simulink library "ammclib_bam_s32k11x"  (Simulink 9.0)
settings: Solver=ode45  StartTime=0.0  StopTime=10.0  RelTol=1e-3
undefined symbols (not defined in the file): f16A1, f16A2, f16B0, f16B1, f16B2, f16C1, f16CC1, f16CC1sc, f16CC1sc_D, f16CC1sc_Q, f16CC1scD, f16CC1scQ, f16CC2, f16CC2sc, f16CC2sc_D, f16CC2sc_Q, f16CC2scD, f16CC2scQ, f16DerivGain, f16EGain, f16FiltCoef, f16HystOff, f16HystOn, f16IGain, f16IntegGain, f16IntegGainFW, f16IntegGainQ, f16Kd, f16Kq, f16Limit, f16LowerLim, f16LowerLimit_D, f16LowerLimit_Q, f16ModIndex, f16OutValOff, f16OutValOn, f16PropGain, f16PropGainFW, f16PropGainQ, f16RampDown, f16RampUp, f16UGain, f16UpperLim, f16UpperLimit, f16UpperLimit_D, f16UpperLimit_Q, f16WIGain, f32A1, f32A2, f32B0, f32B1, f32B2, f32C1, f32CC1, f32CC1sc, f32CC1sc_D, f32CC1sc_Q, f32CC1scD, f32CC1scQ, f32CC2 ... (+71)
(part 1 of 7)
settings Model: Creator=STSP001  LastModifiedBy=nxf35375

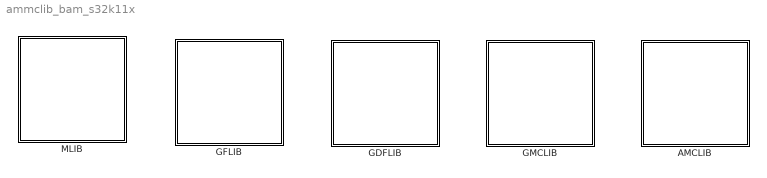
== system ammclib_bam_s32k11x ==
  AMCLIB : Subsystem
  GDFLIB : Subsystem
  GFLIB : Subsystem
  GMCLIB : Subsystem
  MLIB : Subsystem

== system ammclib_bam_s32k11x/AMCLIB ==
  bam_f16 : Subsystem
  bam_f32 : Subsystem

== system ammclib_bam_s32k11x/GDFLIB ==
  bam_f16 : Subsystem
  bam_f32 : Subsystem

== system ammclib_bam_s32k11x/GFLIB ==
  bam_f16 : Subsystem
  bam_f32 : Subsystem

== system ammclib_bam_s32k11x/GMCLIB ==
  bam_f16 : Subsystem
  bam_f32 : Subsystem

== system ammclib_bam_s32k11x/MLIB ==
  bam_f16 : Subsystem
  bam_f32 : Subsystem
  bam_f32f16f16 : Subsystem

== system ammclib_bam_s32k11x/AMCLIB/bam_f16 ==
  AMCLIB_BemfObsrvDQ_F16 : Subsystem  mask(AMCLIB_BemfObsrvDQ_F16){f16IGain=f16IGain, f16UGain=f16UGain, f16WIGain=f16WIGain, f16EGain=f16EGain, s16Shift=s16Shift, f16CC1sc_D=f16CC1sc_D, f16CC1sc_Q=f16CC1sc_Q, f16CC2sc_D=f16CC2sc_D, f16CC2sc_Q=f16CC2sc_Q, f16UpperLimit_D=f16UpperLimit_D, f16UpperLimit_Q=f16UpperLimit_Q, f16LowerLimit_D=f16LowerLimit_D, f16LowerLimit_Q=f16LowerLimit_Q, u16NShift=u16NShift}
      mask help: Bit accurate model of back-EMF observer DQ in 16-bit fixed-point implementation.
      mask init:
      | pos = get_param(gcb, 'Position');width = pos(3) - pos(1); height = pos(4) - pos(2);tX=width/2;tY=height*0.9;
      mask Display: color('black');port_label('input',1,'f16IAB_A');port_label('input',2,'f16IAB_B');port_label('input',3,'f16UAB_A');port_label('input',4,'f16UAB_B');port_label('input',5,'f16Velocity');port_label('input',6,'f16Phase');port_label('output',1,'f16pOutPhaseErr');port_label('output',2,'f16pOutEObsrv_D');port_label('output',3,'f16pOutEObsrv_Q');color('black');disp('AMCLIB_BemfObsrvDQ_F16');color('blue');text(tX,tY, 'BAM', 'horizontalAlignment', 'center');
  AMCLIB_CurrentLoop_F16 : Subsystem  mask(AMCLIB_CurrentLoop_F16){f16CC1scD=f16CC1scD, f16CC2scD=f16CC2scD, u16NShiftD=u16NShiftD, f16CC1scQ=f16CC1scQ, f16CC2scQ=f16CC2scQ, u16NShiftQ=u16NShiftQ}
      mask help: Bit accurate model of the current loop algorithm for a PMSM in 16-bit fixed-point implementation.
      mask init:
      | pos = get_param(gcb, 'Position');width = pos(3) - pos(1); height = pos(4) - pos(2);tX=width/2;tY=height*0.9;
      mask Display: color('black');port_label('input',1,'f16UDcBus');port_label('input',2,'f16IDReq');port_label('input',3,'f16IQReq');port_label('input',4,'f16IDFbck');port_label('input',5,'f16IQFbck');port_label('output',1,'pOutUDReq');port_label('output',2,'pOutUQReq');color('black');disp('AMCLIB_CurrentLoop_F16');color('blue');text(tX,tY, 'BAM', 'horizontalAlignment', 'center');
  AMCLIB_FWSpeedLoop_F16 : Subsystem  mask(AMCLIB_FWSpeedLoop_F16){u16NSamplesW=u16NSamplesW, u16NSamplesFW=u16NSamplesFW, f16PropGainQ=f16PropGainQ, s16PropGainShiftQ=s16PropGainShiftQ, f16IntegGainQ=f16IntegGainQ, s16IntegGainShiftQ=s16IntegGainShiftQ, f16PropGainFW=f16PropGainFW, s16PropGainShiftFW=s16PropGainShiftFW, f16IntegGainFW=f16IntegGainFW, s16IntegGainShiftFW=s16IntegGainShiftFW, f32RampUp=f32RampUp, f32RampDown=f32RampDown}
      mask help: Bit accurate model of the speed loop algorithm with field weakening capability in 16-bit fixed-point implementation.
      mask init:
      | pos = get_param(gcb, 'Position');width = pos(3) - pos(1); height = pos(4) - pos(2);tX=width/2;tY=height*0.9;
      mask Display: color('black');port_label('input',1,'f16VelocityReq');port_label('input',2,'f16VelocityFbck');port_label('input',3,'f16IQFbck');port_label('input',4,'f16UQReq');port_label('input',5,'f16UQLim');port_label('input',6,'f16UpperLimitQ');port_label('input',7,'f16LowerLimitQ');port_label('input',8,'f16UpperLimitFW');port_label('input',9,'f16LowerLimitFW');port_label('output',1,'pOutLimitFlagQ');port_label('output',2,'pOutLimitFlagFW');port_label('output',3,'pOutIDReq');color('black');disp('AMCLIB_FWSpeedLoop_F16');color('blue');text(tX,tY, 'BAM', 'horizontalAlignment', 'center');
  AMCLIB_FW_F16 : Subsystem  mask(AMCLIB_FW_F16){u16NSamplesFW=u16NSamplesFW, f16PropGainFW=f16PropGainFW, s16PropGainShiftFW=s16PropGainShiftFW, f16IntegGainFW=f16IntegGainFW, s16IntegGainShiftFW=s16IntegGainShiftFW}
      mask help: Bit accurate model of the speed loop algorithm with field weakening capability in 16-bit fixed-point implementation.
      mask init:
      | pos = get_param(gcb, 'Position');width = pos(3) - pos(1); height = pos(4) - pos(2);tX=width/2;tY=height*0.9;
      mask Display: color('black');port_label('input',1,'f16ReqAmp');port_label('input',2,'f16VelocityFbck');port_label('input',3,'f16IQFbck');port_label('input',4,'f16UQReq');port_label('input',5,'f16UQLim');port_label('input',6,'f16UpperLimitFW');port_label('input',7,'f16LowerLimitFW');port_label('output',1,'pOutLimitFlagFW');port_label('output',2,'pOutIDReq');color('black');disp('AMCLIB_FW_F16');color('blue');text(tX,tY, 'BAM', 'horizontalAlignment', 'center');
  AMCLIB_SpeedLoop_F16 : Subsystem  mask(AMCLIB_SpeedLoop_F16){u16NSamplesW=u16NSamplesW, f16PropGainQ=f16PropGainQ, s16PropGainShiftQ=s16PropGainShiftQ, f16IntegGainQ=f16IntegGainQ, s16IntegGainShiftQ=s16IntegGainShiftQ, f32RampUp=f32RampUp, f32RampDown=f32RampDown}
      mask help: Bit accurate model of the speed loop algorithm with field weakening capability in 16-bit fixed-point implementation.
      mask init:
      | pos = get_param(gcb, 'Position');width = pos(3) - pos(1); height = pos(4) - pos(2);tX=width/2;tY=height*0.9;
      mask Display: color('black');port_label('input',1,'f16VelocityReq');port_label('input',2,'f16VelocityFbck');port_label('input',3,'f16UpperLimitQ');port_label('input',4,'f16LowerLimitQ');port_label('output',1,'pOutLimitFlagQ');port_label('output',2,'pOutIQReq');color('black');disp('AMCLIB_SpeedLoop_F16');color('blue');text(tX,tY, 'BAM', 'horizontalAlignment', 'center');
  AMCLIB_TrackObsrv_F16 : Subsystem  mask(AMCLIB_TrackObsrv_F16){f16CC1sc=f16CC1sc, f16CC2sc=f16CC2sc, u16NShift=u16NShift, f16C1=f16C1, u16IntegNShift=u16IntegNShift}
      mask help: Bit accurate model of the tracking observer function.
      mask init:
      | pos = get_param(gcb, 'Position');width = pos(3) - pos(1); height = pos(4) - pos(2);tX=width/2;tY=height*0.9;
      mask Display: color('black');port_label('input',1,'f16PhaseErr');port_label('input',2,'f16UpperLimit');port_label('input',3,'f16LowerLimit');port_label('output',1,'f16PosEst');port_label('output',2,'f16VelocityEst');color('black');disp('AMCLIB_TrackObsrv_F16');color('blue');text(tX,tY, 'BAM', 'horizontalAlignment', 'center');

== system ammclib_bam_s32k11x/AMCLIB/bam_f32 ==
  AMCLIB_BemfObsrvDQ_F32 : Subsystem  mask(AMCLIB_BemfObsrvDQ_F32){f32IGain=f32IGain, f32UGain=f32UGain, f32WIGain=f32WIGain, f32EGain=f32EGain, s16Shift=s16Shift, f32CC1sc_D=f32CC1sc_D, f32CC1sc_Q=f32CC1sc_Q, f32CC2sc_D=f32CC2sc_D, f32CC2sc_Q=f32CC2sc_Q, f32UpperLimit_D=f32UpperLimit_D, f32UpperLimit_Q=f32UpperLimit_Q, f32LowerLimit_D=f32LowerLimit_D, f32LowerLimit_Q=f32LowerLimit_Q, u16NShift=u16NShift}
      mask help: Bit accurate model of back-EMF observer DQ in 32-bit fixed-point implementation.
      mask init:
      | pos = get_param(gcb, 'Position');width = pos(3) - pos(1); height = pos(4) - pos(2);tX=width/2;tY=height*0.9;
      mask Display: color('black');port_label('input',1,'f32IAB_A');port_label('input',2,'f32IAB_B');port_label('input',3,'f32UAB_A');port_label('input',4,'f32UAB_B');port_label('input',5,'f32Velocity');port_label('input',6,'f32Phase');port_label('output',1,'f32pOutPhaseErr');port_label('output',2,'f32pOutEObsrv_D');port_label('output',3,'f32pOutEObsrv_Q');color('black');disp('AMCLIB_BemfObsrvDQ_F32');color('blue');text(tX,tY, 'BAM', 'horizontalAlignment', 'center');
  AMCLIB_CurrentLoop_F32 : Subsystem  mask(AMCLIB_CurrentLoop_F32){f32CC1scD=f32CC1scD, f32CC2scD=f32CC2scD, u16NShiftD=u16NShiftD, f32CC1scQ=f32CC1scQ, f32CC2scQ=f32CC2scQ, u16NShiftQ=u16NShiftQ}
      mask help: Bit accurate model of the current loop algorithm for a PMSM in 32-bit fixed-point implementation.
      mask init:
      | pos = get_param(gcb, 'Position');width = pos(3) - pos(1); height = pos(4) - pos(2);tX=width/2;tY=height*0.9;
      mask Display: color('black');port_label('input',1,'f32UDcBus');port_label('input',2,'f32IDReq');port_label('input',3,'f32IQReq');port_label('input',4,'f32IDFbck');port_label('input',5,'f32IQFbck');port_label('output',1,'pOutUDReq');port_label('output',2,'pOutUQReq');color('black');disp('AMCLIB_CurrentLoop_F32');color('blue');text(tX,tY, 'BAM', 'horizontalAlignment', 'center');
  AMCLIB_FWSpeedLoop_F32 : Subsystem  mask(AMCLIB_FWSpeedLoop_F32){u16NSamplesW=u16NSamplesW, u16NSamplesFW=u16NSamplesFW, f32PropGainQ=f32PropGainQ, s16PropGainShiftQ=s16PropGainShiftQ, f32IntegGainQ=f32IntegGainQ, s16IntegGainShiftQ=s16IntegGainShiftQ, f32PropGainFW=f32PropGainFW, s16PropGainShiftFW=s16PropGainShiftFW, f32IntegGainFW=f32IntegGainFW, s16IntegGainShiftFW=s16IntegGainShiftFW, f32RampUp=f32RampUp, f32RampDown=f32RampDown}
      mask help: Bit accurate model of the speed loop algorithm with field weakening capability in 32-bit fixed-point implementation.
      mask init:
      | pos = get_param(gcb, 'Position');width = pos(3) - pos(1); height = pos(4) - pos(2);tX=width/2;tY=height*0.9;
      mask Display: color('black');port_label('input',1,'f32VelocityReq');port_label('input',2,'f32VelocityFbck');port_label('input',3,'f32IQFbck');port_label('input',4,'f32UQReq');port_label('input',5,'f32UQLim');port_label('input',6,'f32UpperLimitQ');port_label('input',7,'f32LowerLimitQ');port_label('input',8,'f32UpperLimitFW');port_label('input',9,'f32LowerLimitFW');port_label('output',1,'pOutLimitFlagQ');port_label('output',2,'pOutLimitFlagFW');port_label('output',3,'pOutIDReq');color('black');disp('AMCLIB_FWSpeedLoop_F32');color('blue');text(tX,tY, 'BAM', 'horizontalAlignment', 'center');
  AMCLIB_FW_F32 : Subsystem  mask(AMCLIB_FW_F32){u16NSamplesFW=u16NSamplesFW, f32PropGainFW=f32PropGainFW, s16PropGainShiftFW=s16PropGainShiftFW, f32IntegGainFW=f32IntegGainFW, s16IntegGainShiftFW=s16IntegGainShiftFW}
      mask help: Bit accurate model of the speed loop algorithm with field weakening capability in 32-bit fixed-point implementation.
      mask init:
      | pos = get_param(gcb, 'Position');width = pos(3) - pos(1); height = pos(4) - pos(2);tX=width/2;tY=height*0.9;
      mask Display: color('black');port_label('input',1,'f32ReqAmp');port_label('input',2,'f32VelocityFbck');port_label('input',3,'f32IQFbck');port_label('input',4,'f32UQReq');port_label('input',5,'f32UQLim');port_label('input',6,'f32UpperLimitFW');port_label('input',7,'f32LowerLimitFW');port_label('output',1,'pOutLimitFlagFW');port_label('output',2,'pOutIDReq');color('black');disp('AMCLIB_FW_F32');color('blue');text(tX,tY, 'BAM', 'horizontalAlignment', 'center');
  AMCLIB_SpeedLoop_F32 : Subsystem  mask(AMCLIB_SpeedLoop_F32){u16NSamplesW=u16NSamplesW, f32PropGainQ=f32PropGainQ, s16PropGainShiftQ=s16PropGainShiftQ, f32IntegGainQ=f32IntegGainQ, s16IntegGainShiftQ=s16IntegGainShiftQ, f32RampUp=f32RampUp, f32RampDown=f32RampDown}
      mask help: Bit accurate model of the speed loop algorithm with field weakening capability in 32-bit fixed-point implementation.
      mask init:
      | pos = get_param(gcb, 'Position');width = pos(3) - pos(1); height = pos(4) - pos(2);tX=width/2;tY=height*0.9;
      mask Display: color('black');port_label('input',1,'f32VelocityReq');port_label('input',2,'f32VelocityFbck');port_label('input',3,'f32UpperLimitQ');port_label('input',4,'f32LowerLimitQ');port_label('output',1,'pOutLimitFlagQ');port_label('output',2,'pOutIQReq');color('black');disp('AMCLIB_SpeedLoop_F32');color('blue');text(tX,tY, 'BAM', 'horizontalAlignment', 'center');
  AMCLIB_TrackObsrv_F32 : Subsystem  mask(AMCLIB_TrackObsrv_F32){f32CC1sc=f32CC1sc, f32CC2sc=f32CC2sc, u16NShift=u16NShift, f32C1=f32C1, u16IntegNShift=u16IntegNShift}
      mask help: Bit accurate model of the tracking observer function.
      mask init:
      | pos = get_param(gcb, 'Position');width = pos(3) - pos(1); height = pos(4) - pos(2);tX=width/2;tY=height*0.9;
      mask Display: color('black');port_label('input',1,'f32PhaseErr');port_label('input',2,'f32UpperLimit');port_label('input',3,'f32LowerLimit');port_label('output',1,'f32PosEst');port_label('output',2,'f32VelocityEst');color('black');disp('AMCLIB_TrackObsrv_F32');color('blue');text(tX,tY, 'BAM', 'horizontalAlignment', 'center');

== system ammclib_bam_s32k11x/GDFLIB/bam_f16 ==
  GDFLIB_FilterFIR_F16 : Subsystem  mask(GDFLIB_FilterFIR_F16){u16Order=u16Order, pf16CoefBuf=pf16CoefBuf}
      mask help: Bit accurate model of FIR filter. All parameters as well as input and output are 16bit integers.
      mask init:
      | pos = get_param(gcb, 'Position');width = pos(3) - pos(1); height = pos(4) - pos(2);tX=width/2;tY=height*0.9;
      mask Help: web(fullfile(mbd_s32k_mc_block_help('s32k11x'), 'S32K11XMCLUG.pdf'), '-browser')
      mask Display:
      | color('black');
      | port_label('input',1,'f16In');
      | port_label('output',1,'f16Out');
      | color('black');
      | disp('GDFLIB_FilterFIR_F16');
      | color('blue');
      | text(tX,tY, 'BAM', 'horizontalAlignment', 'center');
  GDFLIB_FilterIIR1_F16 : Subsystem  mask(GDFLIB_FilterIIR1){f16B0=f16B0, f16B1=f16B1, f16A1=f16A1}
      mask help: Bit accurate model of first order IIR filter. All parameters as well as input and output are 16bit integers.
      mask init:
      | pos = get_param(gcb, 'Position');width = pos(3) - pos(1); height = pos(4) - pos(2);tX=width/2;tY=height*0.9;
      mask Help: web(fullfile(mbd_s32k_mc_block_help('s32k11x'), 'S32K11XMCLUG.pdf'), '-browser')
      mask Display: color('black');port_label('input',1,'f16In');port_label('output',1,'f16Out');color('black');disp('GDFLIB_FilterIIR1_F16');color('blue');text(tX,tY, 'BAM', 'horizontalAlignment', 'center');
  GDFLIB_FilterIIR2_F16 : Subsystem  mask(GDFLIB_FilterIIR2){f16B0=f16B0, f16B1=f16B1, f16B2=f16B2, f16A1=f16A1, f16A2=f16A2}
      mask help: Bit accurate model of direct form I second order IIR filter. All parameters as well as input and output are 16bit integers.
      mask init:
      | pos = get_param(gcb, 'Position');width = pos(3) - pos(1); height = pos(4) - pos(2);tX=width/2;tY=height*0.9;
      mask Help: web(fullfile(mbd_s32k_mc_block_help('s32k11x'), 'S32K11XMCLUG.pdf'), '-browser')
      mask Display: color('black');port_label('input',1,'f16In');port_label('output',1,'f16Out');color('black');disp('GDFLIB_FilterIIR2_F16');color('blue');text(tX,tY, 'BAM', 'horizontalAlignment', 'center');
  GDFLIB_FilterMA_F16 : Subsystem  mask(GDFLIB_FilterMA_F16){u16NSamples=u16NSamples}
      mask help: Bit accurate model of recursive form moving average filter. All parameters as well as input and output are 16bit integers.
      mask init:
      | pos = get_param(gcb, 'Position');width = pos(3) - pos(1); height = pos(4) - pos(2);tX=width/2;tY=height*0.9;
      mask Help: web(fullfile(mbd_s32k_mc_block_help('s32k11x'), 'S32K11XMCLUG.pdf'), '-browser')
      mask Display:
      | color('black');
      | port_label('input',1,'f16In');
      | port_label('output',1,'f16Out');
      | color('black');
      | disp('GDFLIB_FilterMA_F16');
      | color('blue');
      | text(tX,tY, 'BAM', 'horizontalAlignment', 'center');

== system ammclib_bam_s32k11x/GDFLIB/bam_f32 ==
  GDFLIB_FilterFIR_F32 : Subsystem  mask(GDFLIB_FilterFIR_F32){u32Order=u32Order, pf32CoefBuf=pf32CoefBuf}
      mask help: Bit accurate model of FIR filter. All parameters as well as input and output are 32bit integers.
      mask init:
      | pos = get_param(gcb, 'Position');width = pos(3) - pos(1); height = pos(4) - pos(2);tX=width/2;tY=height*0.9;
      mask Help: web(fullfile(mbd_s32k_mc_block_help('s32k11x'), 'S32K11XMCLUG.pdf'), '-browser')
      mask Display:
      | color('black');
      | port_label('input',1,'f32In');
      | port_label('output',1,'f32Out');
      | color('black');
      | disp('GDFLIB_FilterFIR_F32');
      | color('blue');
      | text(tX,tY, 'BAM', 'horizontalAlignment', 'center');
  GDFLIB_FilterIIR1_F32 : Subsystem  mask(GDFLIB_FilterIIR1){f32B0=f32B0, f32B1=f32B1, f32A1=f32A1}
      mask help: Bit accurate model of first order IIR filter. All parameters as well as input and output are 32bit integers.
      mask init:
      | pos = get_param(gcb, 'Position');width = pos(3) - pos(1); height = pos(4) - pos(2);tX=width/2;tY=height*0.9;
      mask Help: web(fullfile(mbd_s32k_mc_block_help('s32k11x'), 'S32K11XMCLUG.pdf'), '-browser')
      mask Display: color('black');port_label('input',1,'f32In');port_label('output',1,'f32Out');color('black');disp('GDFLIB_FilterIIR1_F32');color('blue');text(tX,tY, 'BAM', 'horizontalAlignment', 'center');
  GDFLIB_FilterIIR2_F32 : Subsystem  mask(GDFLIB_FilterIIR2){f32B0=f32B0, f32B1=f32B1, f32B2=f32B2, f32A1=f32A1, f32A2=f32A2}
      mask help: Bit accurate model of direct form I second order IIR filter. All parameters as well as input and output are 32bit integers.
      mask init:
      | pos = get_param(gcb, 'Position');width = pos(3) - pos(1); height = pos(4) - pos(2);tX=width/2;tY=height*0.9;
      mask Help: web(fullfile(mbd_s32k_mc_block_help('s32k11x'), 'S32K11XMCLUG.pdf'), '-browser')
      mask Display: color('black');port_label('input',1,'f32In');port_label('output',1,'f32Out');color('black');disp('GDFLIB_FilterIIR2_F32');color('blue');text(tX,tY, 'BAM', 'horizontalAlignment', 'center');
  GDFLIB_FilterMA_F32 : Subsystem  mask(GDFLIB_FilterMA_F32){u16NSamples=u16NSamples}
      mask help: Bit accurate model of recursive form moving average filter. All parameters as well as input and output are 32bit integers.
      mask init:
      | pos = get_param(gcb, 'Position');width = pos(3) - pos(1); height = pos(4) - pos(2);tX=width/2;tY=height*0.9;
      mask Help: web(fullfile(mbd_s32k_mc_block_help('s32k11x'), 'S32K11XMCLUG.pdf'), '-browser')
      mask Display:
      | color('black');
      | port_label('input',1,'f32In');
      | port_label('output',1,'f32Out');
      | color('black');
      | disp('GDFLIB_FilterMA_F32');
      | color('blue');
      | text(tX,tY, 'BAM', 'horizontalAlignment', 'center');

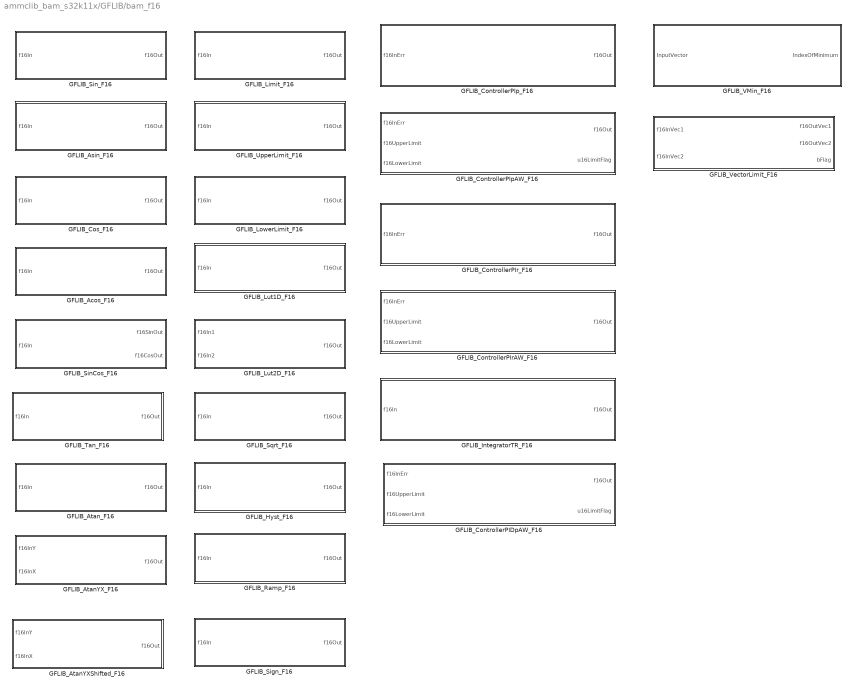
== system ammclib_bam_s32k11x/GFLIB/bam_f16 ==
  GFLIB_Acos_F16 : Subsystem  mask(GFLIB_Acos_F16){}
      mask help: Bit accurate model of GFLIB_Acos function, which computes the acos(fltIn) using the 4th order Taylor polynomial approximation.
      mask init:
      | pos = get_param(gcb, 'Position');width = pos(3) - pos(1); height = pos(4) - pos(2);tX=width/2;tY=height*0.9;
      mask Help: web(fullfile(mbd_s32k_mc_block_help('s32k11x'), 'S32K11XMCLUG.pdf'), '-browser')
      mask Display: color('black');port_label('input',1,'f16In');port_label('output',1,'f16Out');color('black');disp('GFLIB_Acos_F16');color('blue');text(tX,tY, 'BAM', 'horizontalAlignment', 'center');
  GFLIB_Asin_F16 : Subsystem  mask(GFLIB_Asin_F16){}
      mask help: Bit accurate model of GFLIB_Asin function, which computes the asin(f16In) using the 4th order Taylor polynomial approximation.
      mask init:
      | pos = get_param(gcb, 'Position');width = pos(3) - pos(1); height = pos(4) - pos(2);tX=width/2;tY=height*0.9;
      mask Help: web(fullfile(mbd_s32k_mc_block_help('s32k11x'), 'S32K11XMCLUG.pdf'), '-browser')
      mask Display: color('black');port_label('input',1,'f16In');port_label('output',1,'f16Out');color('black');disp('GFLIB_Asin_F16');color('blue');text(tX,tY, 'BAM', 'horizontalAlignment', 'center');
  GFLIB_AtanYXShifted_F16 : Subsystem  mask(GFLIB_AtanYXShifted_F16){Ky=Ky, Kx=Kx, Ny=Ny, Nx=Nx, ThetaAdj=ThetaAdj}
      mask help: Bit accurate model of GFLIB_AtanYXShifted function.
      mask init:
      | pos = get_param(gcb, 'Position');width = pos(3) - pos(1); height = pos(4) - pos(2);tX=width/2;tY=height*0.9;
      mask Help: web(fullfile(mbd_s32k_mc_block_help('s32k11x'), 'S32K11XMCLUG.pdf'), '-browser')
      mask Display: color('black');port_label('input',1,'f16InY');port_label('input',2,'f16InX');port_label('output',1,'f16Out');color('black');disp('GFLIB_AtanYXShifted_F16');color('blue');text(tX,tY, 'BAM', 'horizontalAlignment', 'center');
  GFLIB_AtanYX_F16 : Subsystem  mask(GFLIB_AtanYX_F16){}
      mask help: Bit accurate model of GFLIB_AtanYX function.
      mask init:
      | pos = get_param(gcb, 'Position');width = pos(3) - pos(1); height = pos(4) - pos(2);tX=width/2;tY=height*0.9;
      mask Help: web(fullfile(mbd_s32k_mc_block_help('s32k11x'), 'S32K11XMCLUG.pdf'), '-browser')
      mask Display: color('black');port_label('input',1,'f16InY');port_label('input',2,'f16InX');port_label('output',1,'f16Out');color('black');disp('GFLIB_AtanYX_F16');color('blue');text(tX,tY, 'BAM', 'horizontalAlignment', 'center');
  GFLIB_Atan_F16 : Subsystem  mask(GFLIB_Atan_F16){}
      mask help: Bit accurate model of GFLIB_Atan function, which computes the arctan(f16In) function.
      mask init:
      | pos = get_param(gcb, 'Position');width = pos(3) - pos(1); height = pos(4) - pos(2);tX=width/2;tY=height*0.9;
      mask Help: web(fullfile(mbd_s32k_mc_block_help('s32k11x'), 'S32K11XMCLUG.pdf'), '-browser')
      mask Display: color('black');port_label('input',1,'f16In');port_label('output',1,'f16Out');color('black');disp('GFLIB_Atan_F16');color('blue');text(tX,tY, 'BAM', 'horizontalAlignment', 'center');
  GFLIB_ControllerPIDpAW_F16 : Subsystem  mask(GFLIB_ControllerPIDpAW_F16){f16PropGain=f16PropGain, s16PropGainShift=s16PropGainShift, f16IntegGain=f16IntegGain, s16IntegGainShift=s16IntegGainShift, f16DerivGain=f16DerivGain, s16DerivGainShift=s16DerivGainShift, f16FiltCoef=f16FiltCoef}
      mask help: Bit accurate model of parallel form PID controller. All parameters as well as input and output are 16-bit integers except for s16xxxGainShift parameters which are 16-bit signed integers.
      mask init:
      | pos = get_param(gcb, 'Position');width = pos(3) - pos(1); height = pos(4) - pos(2);tX=width/2;tY=height*0.9;
      mask Display: color('black');port_label('input',1,'f16InErr');port_label('input',2,'f16UpperLimit');port_label('input',3,'f16LowerLimit');port_label('output',1,'f16Out');port_label('output',2,'u16LimitFlag');color('black');disp('GFLIB_ControllerPIDpAW_F16');color('blue');text(tX,tY, 'BAM', 'horizontalAlignment', 'center');
  GFLIB_ControllerPIpAW_F16 : Subsystem  mask(GFLIB_ControllerPIpAW_F16){f16PropGain=f16PropGain, s16PropGainShift=s16PropGainShift, f16IntegGain=f16IntegGain, s16IntegGainShift=s16IntegGainShift}
      mask help: Bit accurate model of parallel form PI controller with anti-windup. All parameters as well as input and output are 16-bit integers except for u16NShift parameter which is 16-bit unsigned integer.
      mask init:
      | pos = get_param(gcb, 'Position');width = pos(3) - pos(1); height = pos(4) - pos(2);tX=width/2;tY=height*0.9;
      mask Help: web(fullfile(mbd_s32k_mc_block_help('s32k11x'), 'S32K11XMCLUG.pdf'), '-browser')
      mask Display: color('black');port_label('input',1,'f16InErr');port_label('input',2,'f16UpperLimit');port_label('input',3,'f16LowerLimit');port_label('output',1,'f16Out');port_label('output',2,'u16LimitFlag');color('black');disp('GFLIB_ControllerPIpAW_F16');color('blue');text(tX,tY, 'BAM', 'horizontalAlignment', 'center');
  GFLIB_ControllerPIp_F16 : Subsystem  mask(GFLIB_ControllerPIp_F16){f16PropGain=f16PropGain, s16PropGainShift=s16PropGainShift, f16IntegGain=f16IntegGain, s16IntegGainShift=s16IntegGainShift}
      mask help: Bit accurate model of parallel form PI controller. All parameters as well as input and output are 16-bit integers except for u16NShift parameter which is 16-bit unsigned integer.
      mask init:
      | pos = get_param(gcb, 'Position');width = pos(3) - pos(1); height = pos(4) - pos(2);tX=width/2;tY=height*0.9;
      mask Help: web(fullfile(mbd_s32k_mc_block_help('s32k11x'), 'S32K11XMCLUG.pdf'), '-browser')
      mask Display:
      | color('black');
      | port_label('input',1,'f16InErr');
      | port_label('output',1,'f16Out');
      | color('black');
      | disp('GFLIB_ControllerPIp_F16');
      | color('blue');
      | text(tX,tY, 'BAM', 'horizontalAlignment', 'center');
  GFLIB_ControllerPIrAW_F16 : Subsystem  mask(GFLIB_ControllerPIrAW_F16){f16CC1=f16CC1, f16CC2=f16CC2, u16NShift=u16NShift}
      mask help: Bit accurate model of reccurent form PI controller with anti-windup. All parameters as well as input and output are 16-bit integers except for u16NShift parameter which is 16-bit unsigned integer.
      mask init:
      | pos = get_param(gcb, 'Position');width = pos(3) - pos(1); height = pos(4) - pos(2);tX=width/2;tY=height*0.9;
      mask Help: web(fullfile(mbd_s32k_mc_block_help('s32k11x'), 'S32K11XMCLUG.pdf'), '-browser')
      mask Display: color('black');port_label('input',1,'f16InErr');port_label('input',2,'f16UpperLimit');port_label('input',3,'f16LowerLimit');port_label('output',1,'f16Out');color('black');disp('GFLIB_ControllerPIrAW_F16');color('blue');text(tX,tY, 'BAM', 'horizontalAlignment', 'center');
  GFLIB_ControllerPIr_F16 : Subsystem  mask(GFLIB_ControllerPIr_F16){f16CC1=f16CC1, f16CC2=f16CC2, u16NShift=u16NShift}
      mask help: Bit accurate model of reccurent form PI controller. All parameters as well as input and output are 16-bit integers except for u16NShift parameter which is 16-bit unsigned integer.
      mask init:
      | pos = get_param(gcb, 'Position');width = pos(3) - pos(1); height = pos(4) - pos(2);tX=width/2;tY=height*0.9;
      mask Help: web(fullfile(mbd_s32k_mc_block_help('s32k11x'), 'S32K11XMCLUG.pdf'), '-browser')
      mask Display:
      | color('black');
      | port_label('input',1,'f16InErr');
      | port_label('output',1,'f16Out');
      | color('black');
      | disp('GFLIB_ControllerPIr_F16');
      | color('blue');
      | text(tX,tY, 'BAM', 'horizontalAlignment', 'center');
  GFLIB_Cos_F16 : Subsystem  mask(GFLIB_Cos_F16){}
      mask help: Bit accurate model of GFLIB_Cos function, which computes the cos(f16In) using the 7th order Taylor polynomial approximation.
      mask init:
      | pos = get_param(gcb, 'Position');width = pos(3) - pos(1); height = pos(4) - pos(2);tX=width/2;tY=height*0.9;
      mask Help: web(fullfile(mbd_s32k_mc_block_help('s32k11x'), 'S32K11XMCLUG.pdf'), '-browser')
      mask Display: color('black');port_label('input',1,'f16In');port_label('output',1,'f16Out');color('black');disp('GFLIB_Cos_F16');color('blue');text(tX,tY, 'BAM', 'horizontalAlignment', 'center');
  GFLIB_Hyst_F16 : Subsystem  mask(GFLIB_Hyst_F16){f16HystOn=f16HystOn, f16HystOff=f16HystOff, f16OutValOn=f16OutValOn, f16OutValOff=f16OutValOff}
      mask help: Bit accurate model of hysteresis function. All parameters as well as input and output are 16-bit integers.
      mask init:
      | pos = get_param(gcb, 'Position');width = pos(3) - pos(1); height = pos(4) - pos(2);tX=width/2;tY=height*0.9;
      mask Help: web(fullfile(mbd_s32k_mc_block_help('s32k11x'), 'S32K11XMCLUG.pdf'), '-browser')
      mask Display: color('black');port_label('input',1,'f16In');port_label('output',1,'f16Out');color('black');disp('GFLIB_Hyst_F16');color('blue');text(tX,tY, 'BAM', 'horizontalAlignment', 'center');
  GFLIB_IntegratorTR_F16 : Subsystem  mask(GFLIB_IntegratorTR_F16){f16C1=f16C1, u16NShift=u16NShift}
      mask help: Bit accurate model of discrete trapezoidal integrator. All parameters as well as input and output are full float range.
      mask init:
      | pos = get_param(gcb, 'Position');width = pos(3) - pos(1); height = pos(4) - pos(2);tX=width/2;tY=height*0.9;
      mask Help: web(fullfile(mbd_s32k_mc_block_help('s32k11x'), 'S32K11XMCLUG.pdf'), '-browser')
      mask Display:
      | color('black');
      | port_label('input',1,'f16In');
      | port_label('output',1,'f16Out');
      | color('black');
      | disp('GFLIB_IntegratorTR_F16');
      | color('blue');
      | text(tX,tY, 'BAM', 'horizontalAlignment', 'center');
  GFLIB_Limit_F16 : Subsystem  mask(GFLIB_Limit){f16UpperLimit=f16UpperLimit, f16LowerLim=f16LowerLim}
      mask help: Bit accurate model of the GFLIB_Limit function.
      mask init:
      | pos = get_param(gcb, 'Position');width = pos(3) - pos(1); height = pos(4) - pos(2);tX=width/2;tY=height*0.9;
      mask Help: web(fullfile(mbd_s32k_mc_block_help('s32k11x'), 'S32K11XMCLUG.pdf'), '-browser')
      mask Display: color('black');port_label('input',1,'f16In');port_label('output',1,'f16Out');color('black');disp('GFLIB_Limit_F16');color('blue');text(tX,tY, 'BAM', 'horizontalAlignment', 'center');
  GFLIB_LowerLimit_F16 : Subsystem  mask(GFLIB_LowerLimit_F16){f16LowerLim=f16LowerLim}
      mask help: Bit accurate model of GFLIB_LowerLimit function.
      mask init:
      | pos = get_param(gcb, 'Position');width = pos(3) - pos(1); height = pos(4) - pos(2);tX=width/2;tY=height*0.9;
      mask Help: web(fullfile(mbd_s32k_mc_block_help('s32k11x'), 'S32K11XMCLUG.pdf'), '-browser')
      mask Display: color('black');port_label('input',1,'f16In');port_label('output',1,'f16Out');color('black');disp('GFLIB_LowerLimit_F16');color('blue');text(tX,tY, 'BAM', 'horizontalAlignment', 'center');
  GFLIB_Lut1D_F16 : Subsystem  mask(GFLIB_Lut1D_F16){u16ShamOffset=u16ShamOffset, pf16Table=pf16Table, s16MidIdx=s16MidIdx}
      mask help: Bit accurate model of Lut1D function.
      mask init:
      | pos = get_param(gcb, 'Position');width = pos(3) - pos(1); height = pos(4) - pos(2);tX=width/2;tY=height*0.9;
      mask Help: web(fullfile(mbd_s32k_mc_block_help('s32k11x'), 'S32K11XMCLUG.pdf'), '-browser')
      mask Display: color('black');port_label('input',1,'f16In');port_label('output',1,'f16Out');color('black');disp('GFLIB_Lut1D_F16');color('blue');text(tX,tY, 'BAM', 'horizontalAlignment', 'center');
  GFLIB_Lut2D_F16 : Subsystem  mask(GFLIB_Lut2D_F16){u16ShamOffset1=u16ShamOffset1, u16ShamOffset2=u16ShamOffset2, pf16Table=pf16Table, s16MidIdx=s16MidIdx}
      mask help: Bit accurate model of Lut2D function.
      mask init:
      | pos = get_param(gcb, 'Position');width = pos(3) - pos(1); height = pos(4) - pos(2);tX=width/2;tY=height*0.9;
      mask Help: web(fullfile(mbd_s32k_mc_block_help('s32k11x'), 'S32K11XMCLUG.pdf'), '-browser')
      mask Display: color('black');port_label('input',1,'f16In1');port_label('input',2,'f16In2');port_label('output',1,'f16Out');color('black');disp('GFLIB_Lut2D_F16');color('blue');text(tX,tY, 'BAM', 'horizontalAlignment', 'center');
  GFLIB_Ramp_F16 : Subsystem  mask(GFLIB_Ramp){f16RampUp=f16RampUp, f16RampDown=f16RampDown}
      mask help: Bit accurate model of ramp function. All parameters as well as input and output are 16bit integers.
      mask init:
      | pos = get_param(gcb, 'Position');width = pos(3) - pos(1); height = pos(4) - pos(2);tX=width/2;tY=height*0.9;
      mask Help: web(fullfile(mbd_s32k_mc_block_help('s32k11x'), 'S32K11XMCLUG.pdf'), '-browser')
      mask Display: color('black');port_label('input',1,'f16In');port_label('output',1,'f16Out');color('black');disp('GFLIB_Ramp_F16');color('blue');text(tX,tY, 'BAM', 'horizontalAlignment', 'center');
  GFLIB_Sign_F16 : Subsystem  mask(GFLIB_Sign_F16){}
      mask help: Bit accurate model of GFLIB_Sign function.
      mask init:
      | pos = get_param(gcb, 'Position');width = pos(3) - pos(1); height = pos(4) - pos(2);tX=width/2;tY=height*0.9;
      mask Help: web(fullfile(mbd_s32k_mc_block_help('s32k11x'), 'S32K11XMCLUG.pdf'), '-browser')
      mask Display: color('black');port_label('input',1,'f16In');port_label('output',1,'f16Out');color('black');disp('GFLIB_Sign_F16');color('blue');text(tX,tY, 'BAM', 'horizontalAlignment', 'center');
  GFLIB_SinCos_F16 : Subsystem  mask(GFLIB_SinCos_F16){}
      mask help: Bit accurate model of GFLIB_SinCos function, which computes the sin(f16In) and cos(f16In) using the 7th order Taylor polynomial approximation.
      mask init:
      | pos = get_param(gcb, 'Position');width = pos(3) - pos(1); height = pos(4) - pos(2);tX=width/2;tY=height*0.9;
      mask Help: web(fullfile(mbd_s32k_mc_block_help('s32k11x'), 'S32K11XMCLUG.pdf'), '-browser')
      mask Display: color('black');port_label('input',1,'f16In');port_label('output',1,'f16SinOut');port_label('output',2,'f16CosOut');color('black');disp('GFLIB_SinCos_F16');color('blue');text(tX,tY, 'BAM', 'horizontalAlignment', 'center');
  GFLIB_Sin_F16 : Subsystem  mask(GFLIB_Sin_F16){}
      mask help: Bit accurate model of GFLIB_Sin function, which computes the sin(f16In) using the 7th order Taylor polynomial approximation.
      mask init:
      | pos = get_param(gcb, 'Position');width = pos(3) - pos(1); height = pos(4) - pos(2);tX=width/2;tY=height*0.9;
      mask Help: web(fullfile(mbd_s32k_mc_block_help('s32k11x'), 'S32K11XMCLUG.pdf'), '-browser')
      mask Display: color('black');port_label('input',1,'f16In');port_label('output',1,'f16Out');color('black');disp('GFLIB_Sin_F16');color('blue');text(tX,tY, 'BAM', 'horizontalAlignment', 'center');
  GFLIB_Sqrt_F16 : Subsystem  mask(GFLIB_Sqrt_F16){}
      mask help: Bit accurate model of GFLIB_Sqrt function, which computes the square root of input value.
      mask init:
      | pos = get_param(gcb, 'Position');width = pos(3) - pos(1); height = pos(4) - pos(2);tX=width/2;tY=height*0.9;
      mask Help: web(fullfile(mbd_s32k_mc_block_help('s32k11x'), 'S32K11XMCLUG.pdf'), '-browser')
      mask Display: color('black');port_label('input',1,'f16In');port_label('output',1,'f16Out');color('black');disp('GFLIB_Sqrt_F16');color('blue');text(tX,tY, 'BAM', 'horizontalAlignment', 'center');
  GFLIB_Tan_F16 : Subsystem  mask(GFLIB_Tan_F16){}
      mask help: Bit accurate model of GFLIB_Tan function, which computes the tan(f16In) function.
      mask init:
      | pos = get_param(gcb, 'Position');width = pos(3) - pos(1); height = pos(4) - pos(2);tX=width/2;tY=height*0.9;
      mask Help: web(fullfile(mbd_s32k_mc_block_help('s32k11x'), 'S32K11XMCLUG.pdf'), '-browser')
      mask Display: color('black');port_label('input',1,'f16In');port_label('output',1,'f16Out');color('black');disp('GFLIB_Tan_F16');color('blue');text(tX,tY, 'BAM', 'horizontalAlignment', 'center');
  GFLIB_UpperLimit_F16 : Subsystem  mask(GFLIB_UpperLimit_F16){f16UpperLim=f16UpperLim}
      mask help: Bit accurate model of GFLIB_UpperLimit function.
      mask init:
      | pos = get_param(gcb, 'Position');width = pos(3) - pos(1); height = pos(4) - pos(2);tX=width/2;tY=height*0.9;
      mask Help: web(fullfile(mbd_s32k_mc_block_help('s32k11x'), 'S32K11XMCLUG.pdf'), '-browser')
      mask Display: color('black');port_label('input',1,'f16In');port_label('output',1,'f16Out');color('black');disp('GFLIB_UpperLimit_F16');color('blue');text(tX,tY, 'BAM', 'horizontalAlignment', 'center');
  GFLIB_VMin_F16 : Subsystem  mask(GFLIB_VMin_F16){N=N}
      mask prompts: N "Vector length"
      mask help: Bit accurate model of GFLIB_VMin function, which finds the index of a vector minimum.
      mask init:
      | pos = get_param(gcb, 'Position');width = pos(3) - pos(1); height = pos(4) - pos(2);tX=width/2;tY=height*0.9;
      mask Help: web(fullfile(mbd_s32k_mc_block_help('s32k11x'), 'S32K11XMCLUG.pdf'), '-browser')
      mask Display: color('black');port_label('input',1,'InputVector');port_label('output',1,'IndexOfMinimum');color('black');disp('GFLIB_VMin_F16');color('blue');text(tX,tY, 'BAM', 'horizontalAlignment', 'center');
  GFLIB_VectorLimit_F16 : Subsystem  mask(GFLIB_VectorLimit){f16Limit=f16Limit}
      mask help: Bit accurate model of the GFLIB_VectorLimit function.
      mask init:
      | pos = get_param(gcb, 'Position');width = pos(3) - pos(1); height = pos(4) - pos(2);tX=width/2;tY=height*0.9;
      mask Help: web(fullfile(mbd_s32k_mc_block_help('s32k11x'), 'S32K11XMCLUG.pdf'), '-browser')
      mask Display: color('black');port_label('input',1,'f16InVec1');port_label('input',2,'f16InVec2');port_label('output',1,'f16OutVec1');port_label('output',2,'f16OutVec2');port_label('output',3,'bFlag');color('black');disp('GFLIB_VectorLimit_F16');color('blue');text(tX,tY, 'BAM', 'horizontalAlignment', 'center');
